simulink model "UKF_Wind_Estimator"  (R2016a)
settings: Solver=FixedStepDiscrete  SolverMode=SingleTasking  StartTime=0.0  StopTime=10.0  RelTol=1e-3
settings Model: Creator=jean-philippecondomines  LastModifiedBy=gautier
settings DataIOCC: LimitDataPoints=on  SaveFormat=Array  SaveOutput=off  SaveTime=off
settings OptimizationCC: DefaultParameterBehavior=Inlined  UseDivisionForNetSlopeComputation=on  UseFloatMulNetSlope=on  DefaultUnderspecifiedDataType=single  UseSpecifiedMinMax=on  InlineInvariantSignals=on  PassReuseOutputArgsAs=Individual arguments  ZeroExternalMemoryAtStartup=off  ZeroInternalMemoryAtStartup=off  NoFixptDivByZeroProtection=on  EfficientFloat2IntCast=on  OptimizeModelRefInitCode=on  LifeSpan=1
settings HardwareCC: ProdBitPerPointer=32  ProdLargestAtomicInteger=Integer  ProdWordSize=32  ProdHWDeviceType=Custom Processor->Custom
settings ModelReferenceCC: PropagateSignalLabelsOutOfModel=off
settings RTWCC: SystemTargetFile=ert.tlc  GenCodeOnly=on  GenerateMakefile=off  TemplateMakefile=ert_default_tmf  GenerateReport=on  BuildConfiguration=Faster Runs  IncludeHyperlinkInReport=on  LaunchReport=on  GenerateTraceInfo=on  GenerateTraceReport=on  GenerateTraceReportSl=on  GenerateTraceReportSf=on  GenerateTraceReportEml=on  GenerateCodeMetricsReport=on  RTWCompilerOptimization=on
settings CodeAppCC: ForceParamTrailComments=on  IgnoreCustomStorageClasses=off  SimulinkDataObjDesc=on  CustomSymbolStrGlobalVar=ukf_$N$M  CustomSymbolStrType=$N$M  CustomSymbolStrFcn=$N$M$F  CustomSymbolStrMacro=$N$M  InsertBlockDesc=on
settings ERTTargetCC: TargetLangStandard=C99 (ISO)  GenerateSampleERTMain=on  IncludeMdlTerminateFcn=off  CombineSignalStateStructs=on  SuppressErrorStatus=on  SupportAbsoluteTime=off  SupportNonFinite=off  SupportComplex=off  InlinedParameterPlacement=NonHierarchical  ERTCustomFileTemplate=example_file_process.tlc  ERTFilePackagingFormat=CompactWithDataFile
settings ConfigComp: CovModelRefEnable=Off

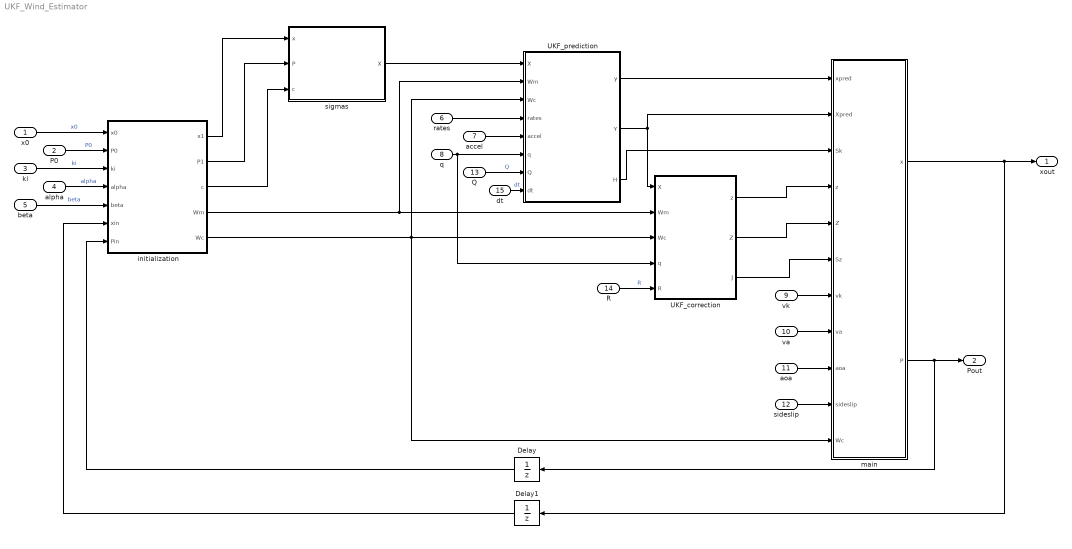
== system UKF_Wind_Estimator ==
  x0 : Inport  OutDataTypeStr=single
  P0 : Inport  Port=2  OutDataTypeStr=single
  ki : Inport  Port=3  OutDataTypeStr=single
  alpha : Inport  Port=4  OutDataTypeStr=single
  beta : Inport  Port=5  OutDataTypeStr=single
  rates : Inport  Port=6  OutDataTypeStr=single
  accel : Inport  Port=7  OutDataTypeStr=single
  q : Inport  Port=8  OutDataTypeStr=single
  vk : Inport  Port=9  OutDataTypeStr=single
  "va " : Inport  Port=10  OutDataTypeStr=single
  aoa : Inport  Port=11  OutDataTypeStr=single
  sideslip : Inport  Port=12  OutDataTypeStr=single
  Q : Inport  Port=13  OutDataTypeStr=single
  R : Inport  Port=14  OutDataTypeStr=single
  dt : Inport  Port=15  OutDataTypeStr=single
  " Delay" : UnitDelay  SampleTime=-1
  " Delay1" : UnitDelay  SampleTime=-1
  UKF_correction : MATLAB Function  TreatAsAtomicUnit=on
  UKF_prediction : MATLAB Function  TreatAsAtomicUnit=on
  initialization : MATLAB Function  TreatAsAtomicUnit=on
  main : MATLAB Function  TreatAsAtomicUnit=on
  sigmas : MATLAB Function  TreatAsAtomicUnit=on
  xout : Outport  OutDataTypeStr=single
  Pout : Outport  Port=2  OutDataTypeStr=single
  wires:
  UKF_correction/1(z) -> main/4(z)
  q/1 -> UKF_correction/4(q), UKF_prediction/6(q)
  beta/1 -> initialization/5(beta)  "beta"
  P0/1 -> initialization/2(P0)  "P0"
  initialization/2(P1) -> sigmas/2(P)
  initialization/5(Wc) -> UKF_correction/3(Wc), main/11(Wc), UKF_prediction/3(Wc)
  vk/1 -> main/7(vk)
  UKF_prediction/3(H) -> main/3(Sk)
  Q/1 -> UKF_prediction/7(Q)  "Q"
  initialization/3(c) -> sigmas/3(c)
  x0/1 -> initialization/1(x0)  "x0"
  sigmas/1(X) -> UKF_prediction/1(X)
  alpha/1 -> initialization/4(alpha)  "alpha"
  UKF_prediction/1(y) -> main/1(xpred)
  initialization/1(x1) -> sigmas/1(x)
  UKF_correction/3(J) -> main/6(Sz)
  dt/1 -> UKF_prediction/8(dt)  "dt"
  main/1(x) -> xout/1, " Delay1"/1
  ki/1 -> initialization/3(ki)  "ki"
  R/1 -> UKF_correction/5(R)  "R"
  UKF_correction/2(Z) -> main/5(Z)
  initialization/4(Wm) -> UKF_prediction/2(Wm), UKF_correction/2(Wm)
  rates/1 -> UKF_prediction/4(rates)
  " Delay"/1 -> initialization/7(Pin)
  main/2(P) -> " Delay"/1, Pout/1
  " Delay1"/1 -> initialization/6(xin)
  accel/1 -> UKF_prediction/5(accel)
  "va "/1 -> main/8(va)
  aoa/1 -> main/9(aoa)
  UKF_prediction/2(Y) -> main/2(Xpred), UKF_correction/1(X)
  sideslip/1 -> main/10(sideslip)

== matlab function UKF_Wind_Estimator/initialization ==
  data: x1 output single size=7; P1 output single size=[7 7]; c output single size=1; x0 input single size=7; Wm output single size=[1 15]; Wc output single size=[1 15]; P0 input single size=[7 7]; ki input single size=1; alpha input single size=1; beta input single size=1; xin input single size=7; Pin input single size=[7 7]
function [x1,P1,c,Wm,Wc] = initialization (x0,P0,ki,alpha,beta,xin,Pin)

%----------------Initialisation---------------------
%P=0*eye(11);
%x=(linspace(0,0,11))';
persistent x
persistent P
%persistent Q
%persistent R

if isempty(P)
    P = (chol(P0))';
else 
    P = Pin;
end

if isempty(x)
    x = x0;
  else 
    x = xin;
end


%%%%%%%%%%%%%%%%--PROGRAMME PRINCIPAL--%%%%%%%%%%%%%%%%

%alpha=0.01;  %10^-1=<alpha=<1 : dispersion des sigma points.
            %Default alpha=0.5;
                            
%ki=0;       %ki>=0 : garantis que la covariance soit semi-definit positive.
            %Default k=0;
                    
%beta=2;     %informations sur les moments d'ordre 3
            %Default beta=2 choix optimal quand la distrib est sup. gaussienne.

%dt=0.02;    %dt pour le Runge-Kutta
                        

%--------Calcul du lambda-----------------

n = single(numel(x));                             %dimension de l'etat

lambda = single(alpha^(2)*(n+ki)-n);                    
c = single(n+lambda);
                                             
%----------------Calcul des ponderations Wm et Wc--------------------

Wm = [lambda/c 0.5/c+zeros(1,2*n)];                                          
Wc = Wm;                                      
Wc(1) = Wc(1)+(1-alpha^(2)+beta);
c = sqrt(c);
x1 = x;
P1 = P;

== matlab function UKF_Wind_Estimator/sigmas ==
  data: x input single size=7; P input single size=[7 7]; c input single size=1; X output single size=[7 15]
%----------------Sigma-point---------------------------

%sigmas points et concatenation : n*(2n+1)
%Inputs : 
%		-States:                                 x 		
%		-Covariance on state :                   P 		
%		-Weighting squate-root 
%		-sigmas-point      (Wm,Wc)               c		
%Outputs :  
%		-Sigmas-points (state) :                 X      	
%----------------------------------------------------
function X = sigmas(x,P,c)

%Covariance with ponderation: A = c * P 
A = single(c*P);

%dimension modification on state 
Y = x(:,ones(1,numel(x)));

%concatenation : X=[x Y+A Y-A]
X = [x Y+A Y-A];

== matlab function UKF_Wind_Estimator/UKF_correction ==
  data: z output single size=[6 1]; Z output single size=[6 15]; X input single size=[7 15]; Wm input single size=[1 15]; J output single size=[6 6]; Wc input single size=[1 15]; q input single size=4; R input single size=[6 6]
%----------------Correction Step-------------------------

%%%%%%%%%%%%%%%%%%%%%%%%%%%%%%%%%%%%%%%%%%%%%%%%%%%%%%%%%%%%%%%%%%%%
%      By Condomines Jean_Philippe - 1 may 2015-   
%                   jp.condomines@gmail.com
%%%%%%%%%%%%%%%%%%%%%%%%%%%%%%%%%%%%%%%%%%%%%%%%%%%%%%%%%%%%%%%%%%%%

%Sigma point and output fonction  h(x_k)
%Inputs : 
%		-Sigmas-points (state)   :                  X      	
%		-Weighting sigmas-points  :                 Wm, Wc 	
%		-Dimension of the measurement vector:       n		
%		-Dimension 2n+1 :                           L  		
%		-Weighting measures (Vk+1):                 R  		
%		-Measures :                                 zk 		
%Outputs :
%		-Sigmas_measures :                          Z 		
%		-Predicted measurement :                    z 		
%		-Covariance on measures :                   J 		
%----------------------------------------------------

function [z,Z,J]=correction(X,Wm,Wc,q,R)

m = 6; % measurement input size
n = 7; % input state size
L = 2*n+1; % sigma state size

%Zeros vector for predicted measures
z = single(zeros(m,1));

%Zeros vector for predicted Sigmas_measures
Z = single(zeros(m,L));

%"for" loop for "measures predicted" and "sigmas_measures" predicted
for k=1:L  

    %non linear function h(x), results : Z(:,k)=[zk+1(0) ... zk+1(2n+1)]
    Z(:,k) = h(X(:,k),q);

    %Predicted measurement
    z=z+Wm(k)*Z(:,k); 
   %  z = Z(:,1);
end
  
%Square-root of R
SR = single(sqrt(R));

%Subtracting of "predicted Sigma measures" et "predicted measurement" with ponderation "Wc"
multi = single(sqrt(Wc(2))*(Z(:,2:L)-z(:,ones(1,L-1))));
 
%Concatenation with the square root of the matrix "R"
tt = single([multi SR]');

%factorization qr, result use in "J" and rest in "Temp" 
%Sz,k+1 = qr{[sqrt(Wc(1)) * [Zk+1(:,2:2n+1)-zk+1]  sqrt(R)]
[~, J] = qr(tt,0);

%Subtracting the first column "zk+1(0)" with all the measurements zk+1 predicted
p = single(Z(:,1)-z(:));

%Test on Wc(1) for cholesky factorization : Cholupdate{Sz,k+1,p,Wc(0)} 
if (Wc(1) < 0) 
        J = single(chol(J'*J-((((-1*Wc(1))^(1/4))*p)*(((-1*Wc(1))^(1/4))*p)'))); 
    else 
        J = single(chol(J'*J+((Wc(1)^(1/4))*p)*((Wc(1)^(1/4))*p)'));    
end 
 
%Transposition to have a lower triangular matrix
J = J';

== matlab function UKF_Wind_Estimator/UKF_prediction ==
  data: y output single size=[7 1]; Y output single size=[7 15]; X input single size=[7 15]; Wm input single size=[1 15]; H output single size=[7 7]; Wc input single size=[1 15]; rates input single size=3; accel input single size=3; q input size=4; Q input single size=[7 7]; dt input single size=1
%----------------Prediction Step-------------------------

%Sigma point and model fonction f(x,u)
%Inputs : 
%		-Sigmas-points (state) :                X      	
%		-Weighting sigmas-points  :             Wm, Wc 	
%		-Command input	 :                      omega, a   
%		-Dimension vector state:                n		
%		-Integration step :                     dt		
%		-Dimension 2n+1 :                       L  		
%		-Weighting state (Wk) :                 Q  		
%Outputs :
%		-Predicted state:                       y 		
%		-Sigmas_state   :                       Y 		
%		-Covariance on state :                  H
%----------------------------------------------------
%----------------Prediction-------------------------
%description :
%Output : SigmaX(k+1) et xmoy(k+1)
%
function [y,Y,H] = prediction(X,Wm,Wc,rates,accel,q,Q,dt)

n = 7; % input state size
L = 2*n+1; % sigma state size

y = single(zeros(n,1));
Y = single(zeros(n,L));

u = [rates', accel'];
for k=1:L  
    Y(:,k) = single(RungeKutta(X(:,k),dt,u,q));%non linear function
    y=y+Wm(k)*Y(:,k);                    %predicted vector on the state
    %y = Y(:,1);
end
 
SQ = single(sqrt(Q));                              %square-root of R
 
multi = single(sqrt(Wc(2))*(Y(:,2:L)-y(:,ones(1,L-1))));
 
tt = [multi SQ]';                          %33*11=>[11*22 11*11]
 
[~, H] = qr(tt,0);                   
 
p = single(Y(:,1)-y(:));
 
if (Wc(1) < 0) 
        H = single(chol(H'*H-((((-1*Wc(1))^(1/4))*p)*(((-1*Wc(1))^(1/4))*p)'))); 
    else 
        H = single(chol(H'*H+((Wc(1)^(1/4))*p)*((Wc(1)^(1/4))*p)'));   
end

== matlab function UKF_Wind_Estimator/main ==
  data: x output single size=[7 1]; P output single size=[7 7]; xpred input single size=[7 1]; Xpred input single size=[7 15]; Sk input single size=[7 7]; z input single size=[6 1]; Z input single size=[6 15]; Sz input single size=[6 6]; vk input single size=3; va input single size=1; aoa input single size=1; sideslip input single size=1; Wc input single size=[1 15]
function [x,P] = main(xpred,Xpred,Sk,z,Z,Sz,vk,va,aoa,sideslip,Wc)

m = 6; % measurement input size
n = 7; % input state size
L = 2*n+1; % sigma state size

zk = [vk', va, aoa, sideslip];

Pxz = (Xpred(:,1:L)-xpred(:,ones(1,L)))*diag(Wc)*(Z(:,1:L)-z(:,ones(1,L)))';
 
%Kalman gain : (Pxz/Sz')/Sz
%Caution "/" is least squares root  for "Ax = b"
K = (Pxz/(Sz)')/Sz;

%Predicted state with Kalman gain "K" : x = xpred + K * (zk - z)
x = xpred + K * (zk' - z);

%Quaternion normalisation
%x(1:4)=normalQ(x(1:4)');

%Cholesky factorization : U = K * Sz   
U = K * Sz;
 
%"for" loop for cholesky factorization
for k=1:m
Sk = chol((Sk'*Sk)-U(:,k)*U(:,k)');
end
 
%"Sk" in "P" and Transpose of "P"
P = Sk';

%SqrtP = sqrt(diag(Sk*Sk'));
